simulink model "event_ex"  (R2022b)
settings: Solver=ode1  StartTime=0.0  StopTime=60  FixedStep=0.01  RelTol=1e-3
libraries: simulink x1
settings Model: Creator=user  LastModifiedBy=user

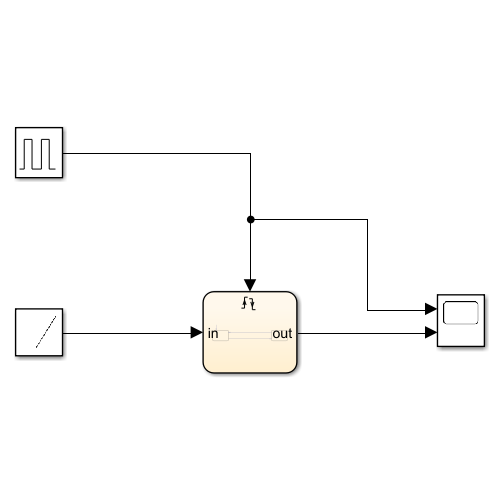
[thumbnail: Simulink's stored preview of the top-level diagram]
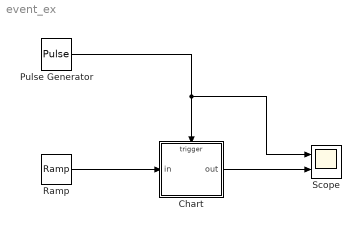
== system event_ex ==
  Chart : Stateflow chart  TreatAsAtomicUnit=on
  Pulse Generator : DiscretePulseGenerator  PulseType=Time based  Period=4  PulseWidth=50
  Ramp : simulink/Sources/Ramp  slope=1  start=0  InitialOutput=0
  Scope : Scope  NumInputPorts=2
  wires:
  Pulse Generator/1 -> Scope/1, Chart/Trigger
  Ramp/1 -> Chart/1(in)
  Chart/1(out) -> Scope/2

== stateflow chart event_ex/Chart ==
  state POS
    en:
    out = in;
  state NEG
    out = -in;
  (default) -> POS
  NEG -> POS : E
  POS -> NEG : E
  data: in input; out output
  events: E input EITHER_EDGE_EVENT
